simulink library "lib_park_transform"  (R2023a)
settings: Solver=VariableStepAuto  StartTime=0.0  StopTime=10.0  RelTol=1e-3
libraries: lib_trigonometric_function x2
settings Model: Creator=cav2ofo  LastModifiedBy=lenovo
settings OptimizationCC: ReuseModelBlockBuffer=off

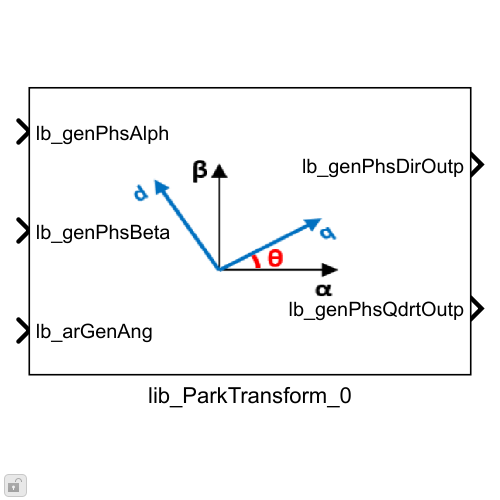
[thumbnail: Simulink's stored preview of the top-level diagram]
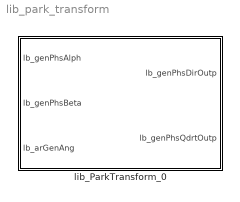
== system lib_park_transform ==
  lib_ParkTransform_0 : Subsystem  VariantControl=ClarkTransf_MIL_flo  mask{lb_parSelRotFrmeAxis=d-axis}
      mask prompts: lb_parSelRotFrmeAxis "Select an axis align:"
      mask init:
      | switch lb_parSelRotFrmeAxis 
      |     case 'd-axis'
      |         set_param([gcb,'/vss_AxisAlignmentVariant'],'LabelModeActiveChoice','lb_parDirToAlphModeLbl');
      |     case 'q-axis'
      |         set_param([gcb,'/vss_AxisAlignmentVariant'],'LabelModeActiveChoice','lb_parQdrtToAlphModeLbl');
      | end
      mask TypeOptions lb_parSelRotFrmeAxis: d-axis | q-axis
      mask DialogControl DescGroupVar Prompt: Park Transform
      mask DialogControl DescTextVar Prompt: VHIT Control Library
      mask DialogControl clarkeDesc Prompt: This block performs Park transformation on stationary reference frame (alpha-beta) inputs into ratating reference frame (d-q) outputs.
      mask DialogControl blockParam Prompt: Block Parameters
      mask DialogControl Control2 Prompt: By default aligns d-axis. Select q-axis from the following list.
      mask Display: image('ParkTransf.PNG'); % Use "Edit Image" on toolstrip to change.

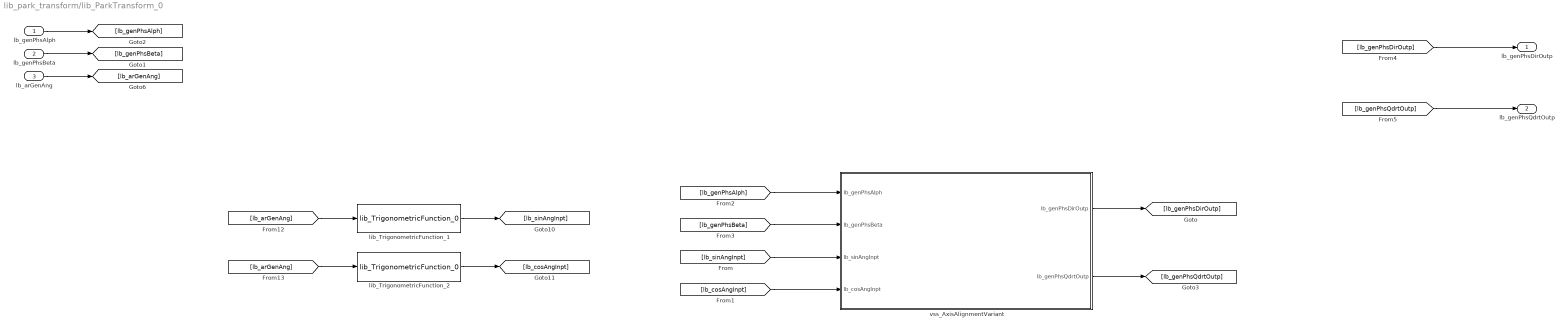
== system lib_park_transform/lib_ParkTransform_0 ==
  lb_genPhsAlph : Inport
  lb_genPhsBeta : Inport  Port=2
  lb_arGenAng : Inport  Port=3
  lib_TrigonometricFunction_1 : lib_trigonometric_function/lib_TrigonometricFunction_0  lb_parSelSigType=Sine  lb_parLktSizeStr=1024  lb_parOutpDataType=fixdt(1,16,2^-14,0)
  lib_TrigonometricFunction_2 : lib_trigonometric_function/lib_TrigonometricFunction_0  lb_parSelSigType=Cosine  lb_parLktSizeStr=1024  lb_parOutpDataType=fixdt(1,16,2^-14,0)
  vss_AxisAlignmentVariant : Subsystem  Variant=on  VariantControlMode=label  VariantControl=Choice  LabelModeActiveChoice=lb_parDirToAlphModeLbl
  lb_genPhsDirOutp : Outport  VectorParamsAs1DForOutWhenUnconnected=off
  lb_genPhsQdrtOutp : Outport  Port=2  VectorParamsAs1DForOutWhenUnconnected=off
  wires:
  lb_arGenAng/1 -> [lb_arGenAng]
  lb_genPhsBeta/1 -> [lb_genPhsBeta]
  lb_genPhsAlph/1 -> [lb_genPhsAlph]
  [lb_genPhsQdrtOutp] -> lb_genPhsQdrtOutp/1
  [lb_genPhsDirOutp] -> lb_genPhsDirOutp/1
  [lb_arGenAng] -> lib_TrigonometricFunction_2/1
  [lb_arGenAng] -> lib_TrigonometricFunction_1/1
  lib_TrigonometricFunction_2/1 -> [lb_cosAngInpt]
  lib_TrigonometricFunction_1/1 -> [lb_sinAngInpt]
  [lb_sinAngInpt] -> vss_AxisAlignmentVariant/3(lb_sinAngInpt)
  [lb_cosAngInpt] -> vss_AxisAlignmentVariant/4(lb_cosAngInpt)
  [lb_genPhsAlph] -> vss_AxisAlignmentVariant/1(lb_genPhsAlph)
  [lb_genPhsBeta] -> vss_AxisAlignmentVariant/2(lb_genPhsBeta)
  vss_AxisAlignmentVariant/1(lb_genPhsDirOutp) -> [lb_genPhsDirOutp]
  vss_AxisAlignmentVariant/2(lb_genPhsQdrtOutp) -> [lb_genPhsQdrtOutp]

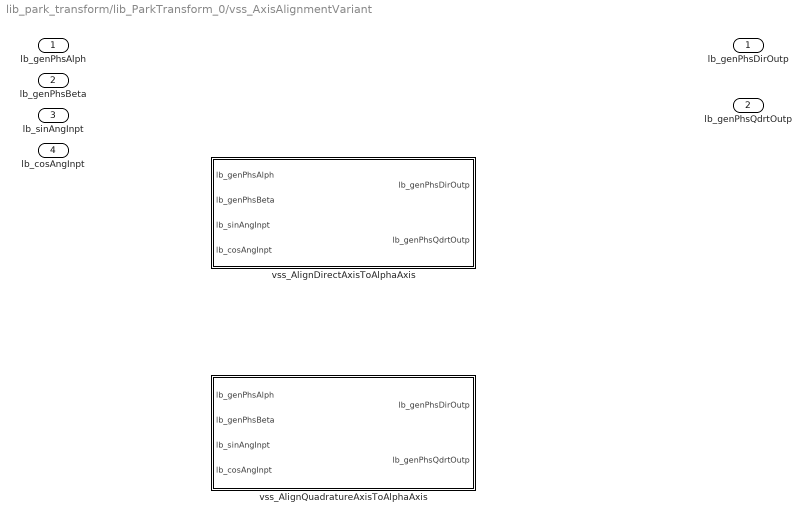
== system lib_park_transform/lib_ParkTransform_0/vss_AxisAlignmentVariant ==
  lb_genPhsAlph : Inport
  lb_genPhsBeta : Inport  Port=2
  lb_sinAngInpt : Inport  Port=3
  lb_cosAngInpt : Inport  Port=4
  vss_AlignDirectAxisToAlphaAxis : Subsystem  VariantControl=lb_parDirToAlphModeLbl
  vss_AlignQuadratureAxisToAlphaAxis : Subsystem  VariantControl=lb_parQdrtToAlphModeLbl
  lb_genPhsDirOutp : Outport  VectorParamsAs1DForOutWhenUnconnected=off
  lb_genPhsQdrtOutp : Outport  Port=2  VectorParamsAs1DForOutWhenUnconnected=off

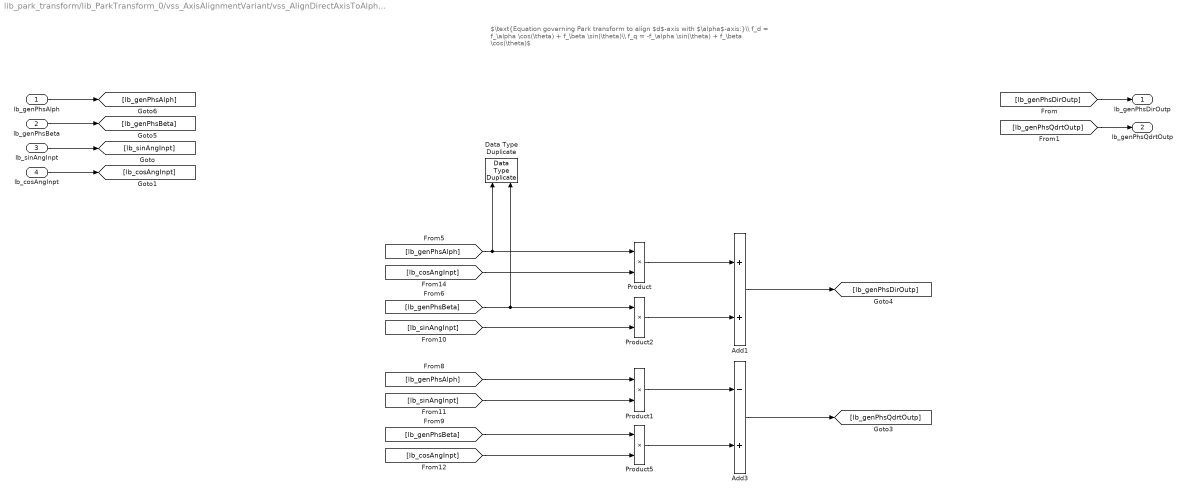
== system lib_park_transform/lib_ParkTransform_0/vss_AxisAlignmentVariant/vss_AlignDirectAxisToAlphaAxis ==
  note: $\text{Equation governing Park transform to align $d$-axis with $\alpha$-axis:}\\ f_d = f_\alpha \cos(\theta) + f_\beta \sin(\theta)\\ f_q = -f_\alpha \sin(\theta) + f_\beta \cos(\theta)$
  lb_genPhsAlph : Inport
  lb_genPhsBeta : Inport  Port=2
  lb_sinAngInpt : Inport  Port=3
  lb_cosAngInpt : Inport  Port=4
  Add1 : Sum  RndMeth=Simplest  OutDataTypeStr=Inherit: Same as first input
  Add3 : Sum  Inputs=-+  RndMeth=Simplest  OutDataTypeStr=Inherit: Same as first input
  Data Type Duplicate : DataTypeDuplicate
  Product{,1..2,5} (4 alike) : Product  RndMeth=Simplest  OutDataTypeStr=Inherit: Same as first input
  lb_genPhsDirOutp : Outport  VectorParamsAs1DForOutWhenUnconnected=off
  lb_genPhsQdrtOutp : Outport  Port=2  VectorParamsAs1DForOutWhenUnconnected=off
  wires:
  lb_cosAngInpt/1 -> [lb_cosAngInpt]
  [lb_cosAngInpt] -> Product/2
  lb_genPhsAlph/1 -> [lb_genPhsAlph]
  [lb_genPhsAlph] -> Product1/1
  Product5/1 -> Add3/2
  [lb_genPhsBeta] -> Product5/1
  lb_sinAngInpt/1 -> [lb_sinAngInpt]
  [lb_genPhsAlph] -> Product/1, Data Type Duplicate/1
  Product/1 -> Add1/1
  [lb_genPhsDirOutp] -> lb_genPhsDirOutp/1
  lb_genPhsBeta/1 -> [lb_genPhsBeta]
  [lb_genPhsBeta] -> Product2/1, Data Type Duplicate/2
  [lb_sinAngInpt] -> Product2/2
  [lb_genPhsQdrtOutp] -> lb_genPhsQdrtOutp/1
  Product1/1 -> Add3/1
  Add1/1 -> [lb_genPhsDirOutp]
  Add3/1 -> [lb_genPhsQdrtOutp]
  [lb_cosAngInpt] -> Product5/2
  Product2/1 -> Add1/2
  [lb_sinAngInpt] -> Product1/2

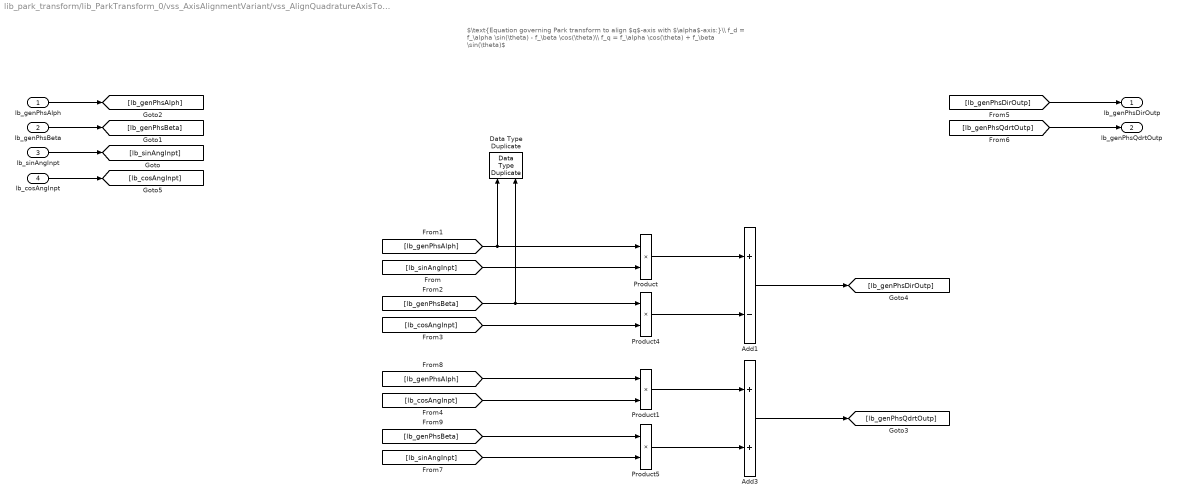
== system lib_park_transform/lib_ParkTransform_0/vss_AxisAlignmentVariant/vss_AlignQuadratureAxisToAlphaAxis ==
  note: $\text{Equation governing Park transform to align $q$-axis with $\alpha$-axis:}\\ f_d = f_\alpha \sin(\theta) - f_\beta \cos(\theta)\\ f_q = f_\alpha \cos(\theta) + f_\beta \sin(\theta)$
  lb_genPhsAlph : Inport
  lb_genPhsBeta : Inport  Port=2
  lb_sinAngInpt : Inport  Port=3
  lb_cosAngInpt : Inport  Port=4
  Add1 : Sum  Inputs=+-  RndMeth=Simplest  OutDataTypeStr=Inherit: Same as first input
  Add3 : Sum  RndMeth=Simplest  OutDataTypeStr=Inherit: Same as first input
  Data Type Duplicate : DataTypeDuplicate
  Product{,1,4..5} (4 alike) : Product  RndMeth=Simplest  OutDataTypeStr=Inherit: Same as first input
  lb_genPhsDirOutp : Outport  VectorParamsAs1DForOutWhenUnconnected=off
  lb_genPhsQdrtOutp : Outport  Port=2  VectorParamsAs1DForOutWhenUnconnected=off
  wires:
  Product/1 -> Add1/1
  Add1/1 -> [lb_genPhsDirOutp]
  [lb_sinAngInpt] -> Product5/2
  [lb_genPhsBeta] -> Product5/1
  Product1/1 -> Add3/1
  lb_genPhsBeta/1 -> [lb_genPhsBeta]
  Product5/1 -> Add3/2
  lb_cosAngInpt/1 -> [lb_cosAngInpt]
  [lb_cosAngInpt] -> Product1/2
  [lb_genPhsAlph] -> Data Type Duplicate/1, Product/1
  [lb_genPhsBeta] -> Product4/1, Data Type Duplicate/2
  [lb_genPhsAlph] -> Product1/1
  Product4/1 -> Add1/2
  [lb_genPhsQdrtOutp] -> lb_genPhsQdrtOutp/1
  [lb_cosAngInpt] -> Product4/2
  [lb_genPhsDirOutp] -> lb_genPhsDirOutp/1
  [lb_sinAngInpt] -> Product/2
  lb_genPhsAlph/1 -> [lb_genPhsAlph]
  lb_sinAngInpt/1 -> [lb_sinAngInpt]
  Add3/1 -> [lb_genPhsQdrtOutp]
